simulink model "est_project_cmsd"  (R2022b)
settings: Solver=ode23  StartTime=0.0  StopTime=50  FixedStep=1e-4  MaxStep=0.1  RelTol=1e-6
values from neighbouring files (symbols this model uses):
  A = [0 0 1 0 ... (first row only)    [cmsd_script.m]
  B = [0,0 ... (first row only)    [cmsd_script.m]
  C = [1 0 0 0 ... (first row only)    [cmsd_script.m]
  delta1 = 1/10    (= 0.1)    [cmsd_nonlinear_discrete.m]    (also in cmsd_script.m)
  delta2 = 1/5    (= 0.2)    [cmsd_nonlinear_discrete.m]    (also in cmsd_script.m)
  F = T*A-K1*C    [cmsd_script.m]
  K = place(A,B,[-3,-3,-4,-4])    [cmsd_script.m]
  k1 = 2/5    (= 0.4)    [cmsd_nonlinear_discrete.m]    (also in cmsd_script.m)
  k2 = 1    [cmsd_nonlinear_discrete.m]    (also in cmsd_script.m)
  L = place(A',C',[-10,-10,-20,-20])'    [cmsd_script.m]
  m1 = 1    [cmsd_nonlinear_discrete.m]    (also in cmsd_script.m)
  m2 = 2    [cmsd_nonlinear_discrete.m]    (also in cmsd_script.m)
  miu1 = 1/6    (= 0.166666666667)    [cmsd_nonlinear_discrete.m]    (also in cmsd_script.m)
  miu2 = 1/10    (= 0.1)    [cmsd_nonlinear_discrete.m]    (also in cmsd_script.m)
settings Model: Creator=Alex  LastModifiedBy=Alex

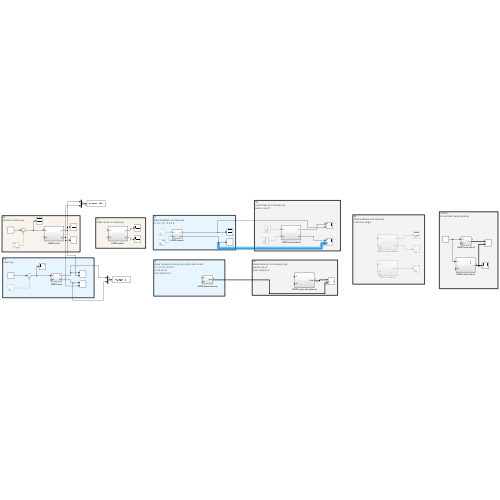
[thumbnail: Simulink's stored preview of the top-level diagram]
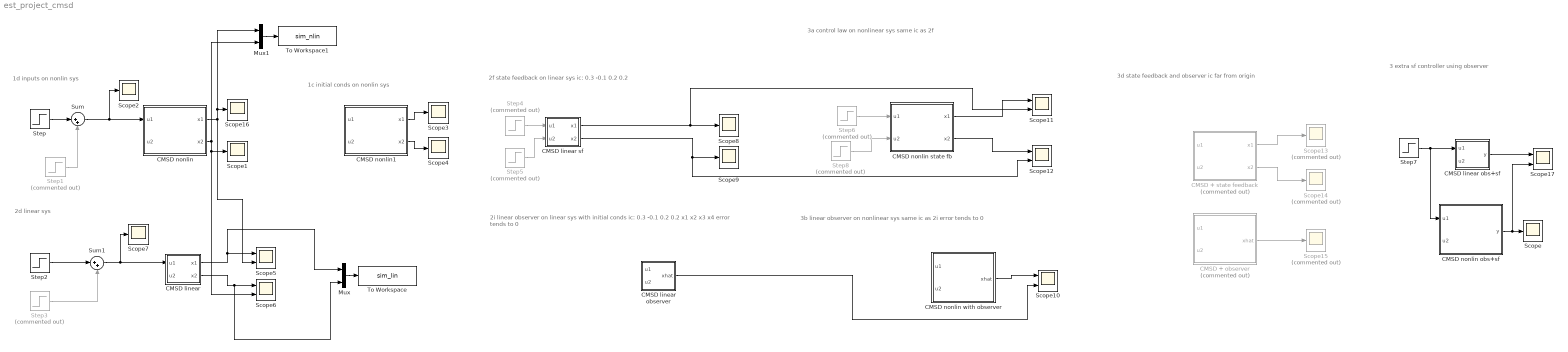
== system est_project_cmsd ==
  note: 3 extra
      | sf controller using observer
  note: 3d
      | state feedback and observer
      | ic far from origin
  note: 3b
      | linear observer on nonlinear sys
      | same ic as 2i
      | error tends to 0
  note: 3a
      | control law on nonlinear sys
      | same ic as 2f
  note: 2i
      | linear observer on linear sys with initial conds
      | ic: 0.3 -0.1 0.2 0.2
      | x1 x2 x3 x4
      | error tends to 0
  note: 2f
      | state feedback on linear sys
      | ic: 0.3 -0.1  0.2 0.2
  note: 2d
      | linear sys
  note: 1d
      | inputs on nonlin sys
  note: 1c
      | initial conds on nonlin sys
  CMSD + observer : Subsystem  Commented=on
  CMSD + state feedback : Subsystem  Commented=on
  CMSD linear : Subsystem
  CMSD linear obs+sf : Subsystem
  CMSD linear observer : Subsystem
  CMSD linear sf : Subsystem
  CMSD nonlin : Subsystem
  CMSD nonlin obs+sf : Subsystem
  CMSD nonlin state fb : Subsystem
  CMSD nonlin with observer : Subsystem
  CMSD nonlin1 : Subsystem
  Mux : Mux  Inputs=2
  Mux1 : Mux  Inputs=2
  Scope{,1..4,7..9,16} (9 alike) : Scope
  Scope{5..6,10..12,17} (6 alike) : Scope  NumInputPorts=2
  Scope13 : Scope  Commented=on
  Scope14 : Scope  Commented=on
  Scope15 : Scope  Commented=on
  Step : Step  Time=0  After=0.1  SampleTime=0
  Step1 : Step  Commented=on  Time=2  After=-0.1  SampleTime=0
  Step2 : Step  Time=0  After=0.1  SampleTime=0
  Step3 : Step  Commented=on  Time=2  After=-0.1  SampleTime=0
  Step4 : Step  Commented=on  SampleTime=0
  Step5 : Step  Commented=on  After=0.2  SampleTime=0
  Step6 : Step  Commented=on  SampleTime=0
  Step7 : Step  After=5  SampleTime=0
  Step8 : Step  Commented=on  After=0.2  SampleTime=0
  Sum : Sum  Inputs=|++
  Sum1 : Sum  Inputs=|++
  To Workspace : ToWorkspace  VariableName=sim_lin  SampleTime=-1
  To Workspace1 : ToWorkspace  VariableName=sim_nlin  SampleTime=-1
  wires:
  Step/1 -> Sum/1
  Step1/1 -> Sum/2
  Sum/1 -> Scope2/1, CMSD nonlin/1(u1)
  CMSD nonlin1/2(x2) -> Scope4/1
  CMSD nonlin1/1(x1) -> Scope3/1
  Sum1/1 -> Scope7/1, CMSD linear/1(u1)
  Step3/1 -> Sum1/2
  Step2/1 -> Sum1/1
  CMSD linear sf/2(x2) -> Scope12/2, Scope9/1
  CMSD linear sf/1(x1) -> Scope11/2, Scope8/1
  CMSD nonlin state fb/1(x1) -> Scope11/1
  CMSD nonlin state fb/2(x2) -> Scope12/1
  CMSD nonlin with observer/1(xhat) -> Scope10/1
  CMSD linear observer/1(xhat) -> Scope10/2
  CMSD + state feedback/1(x1) -> Scope13/1
  CMSD + state feedback/2(x2) -> Scope14/1
  CMSD + observer/1(xhat) -> Scope15/1
  Step4/1 -> CMSD linear sf/1(u1)
  Step5/1 -> CMSD linear sf/2(u2)
  Step6/1 -> CMSD nonlin state fb/1(u1)
  CMSD linear/1(x1) -> Mux/1, Scope5/1
  CMSD nonlin/1(x1) -> Mux1/1, Scope16/1, Scope5/2
  CMSD linear/2(x2) -> Mux/2, Scope6/1
  CMSD nonlin/2(x2) -> Mux1/2, Scope1/1, Scope6/2
  CMSD nonlin obs+sf/1(y) -> Scope17/2, Scope/1
  CMSD linear obs+sf/1(y) -> Scope17/1
  Step7/1 -> CMSD nonlin obs+sf/1(u1), CMSD linear obs+sf/1(u1)
  Step8/1 -> CMSD nonlin state fb/2(u2)
  Mux/1 -> To Workspace/1
  Mux1/1 -> To Workspace1/1

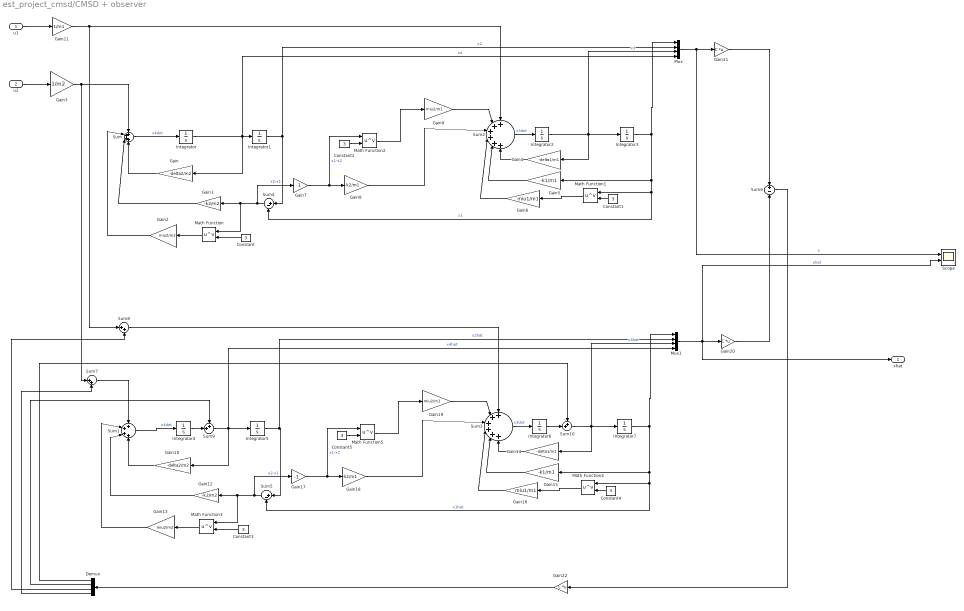
== system est_project_cmsd/CMSD + observer ==
  u1 : Inport
  u2 : Inport  Port=2
  Constant{,1..5} (6 alike) : Constant  Value=3
  Demux : Demux
  Gain : Gain  Gain=-delta2/m2
  Gain1 : Gain  Gain=-k2/m2
  Gain10 : Gain  Gain=-delta2/m2
  Gain11 : Gain  Gain=1/m1
  Gain12 : Gain  Gain=-k2/m2
  Gain13 : Gain  Gain=miu2/m2
  Gain14 : Gain  Gain=-delta1/m1
  Gain15 : Gain  Gain=-k1/m1
  Gain16 : Gain  Gain=miu1/m1
  Gain17 : Gain  Gain=-1
  Gain18 : Gain  Gain=-k2/m1
  Gain19 : Gain  Gain=miu2/m1
  Gain2 : Gain  Gain=miu2/m2
  Gain20 : Gain  Gain=C  Multiplication=Matrix(K*u)
  Gain21 : Gain  Gain=C  Multiplication=Matrix(K*u)
  Gain22 : Gain  Gain=L  Multiplication=Matrix(K*u)
  Gain3 : Gain  Gain=1/m2
  Gain4 : Gain  Gain=-delta1/m1
  Gain5 : Gain  Gain=-k1/m1
  Gain6 : Gain  Gain=miu1/m1
  Gain7 : Gain  Gain=-1
  Gain8 : Gain  Gain=-k2/m1
  Gain9 : Gain  Gain=miu2/m1
  Integrator : Integrator  InitialCondition=0.7
  Integrator1 : Integrator  InitialCondition=-0.6
  Integrator2 : Integrator  InitialCondition=-0.7
  Integrator3 : Integrator  InitialCondition=0.5
  Integrator{4..7} (4 alike) : Integrator
  Math Function{,1..5} (6 alike) : Math  Operator=pow
  Mux : Mux
  Mux1 : Mux
  Scope : Scope  NumInputPorts=2
  Sum : Sum  Inputs=++++
  Sum1 : Sum  Inputs=++++
  Sum10 : Sum  Inputs=++|
  Sum2 : Sum  Inputs=++++++
  Sum3 : Sum  Inputs=++++++
  Sum4 : Sum  Inputs=|+-
  Sum5 : Sum  Inputs=|+-
  Sum6 : Sum  Inputs=+-
  Sum7 : Sum  Inputs=|++
  Sum8 : Sum  Inputs=|++
  Sum9 : Sum  Inputs=++|
  xhat : Outport
  wires:
  Demux/1 -> Sum10/1
  Sum10/1 -> Integrator7/1, Gain14/1, Mux1/3  "x3hat"
  Integrator6/1 -> Sum10/2
  Demux/2 -> Sum9/1
  Sum9/1 -> Integrator5/1, Gain10/1, Mux1/4  "x4hat"
  Integrator4/1 -> Sum9/2
  Demux/3 -> Sum8/2
  Demux/4 -> Sum7/2
  Sum8/1 -> Sum3/1
  Sum7/1 -> Sum1/1
  Gain22/1 -> Demux/1
  Sum6/1 -> Gain22/1
  Gain21/1 -> Sum6/1
  Gain20/1 -> Sum6/2
  Mux1/1 -> Gain20/1, Scope/2, xhat/1  "xhat"
  Gain14/1 -> Sum3/6
  Sum5/1 -> Gain17/1, Math Function3/1, Gain12/1  "x2-x1"
  Integrator7/1 -> Sum5/2, Math Function4/1, Gain15/1, Mux1/1  "x1hat"
  Gain18/1 -> Sum3/3
  Gain17/1 -> Math Function5/1, Gain18/1  "x1-x2"
  Math Function5/1 -> Gain19/1
  Gain15/1 -> Sum3/5
  Gain12/1 -> Sum1/3
  Constant5/1 -> Math Function5/2
  Gain19/1 -> Sum3/2
  Sum1/1 -> Integrator4/1  "x4dot"
  Math Function4/1 -> Gain16/1
  Gain10/1 -> Sum1/4
  Gain13/1 -> Sum1/2
  Integrator5/1 -> Mux1/2, Sum5/1  "x2hat"
  Constant3/1 -> Math Function3/2
  Math Function3/1 -> Gain13/1
  Gain16/1 -> Sum3/4
  Sum3/1 -> Integrator6/1  "x3dot"
  Constant4/1 -> Math Function4/2
  Gain11/1 -> Sum2/1, Sum8/1
  Constant1/1 -> Math Function1/2
  Sum2/1 -> Integrator2/1  "x3dot"
  u2/1 -> Gain3/1
  Gain6/1 -> Sum2/4
  Integrator2/1 -> Mux/3, Integrator3/1, Gain4/1  "x3"
  Math Function/1 -> Gain2/1
  Constant/1 -> Math Function/2
  Integrator1/1 -> Sum4/1, Mux/2  "x2"
  Gain2/1 -> Sum/2
  Gain/1 -> Sum/4
  Math Function1/1 -> Gain6/1
  Sum/1 -> Integrator/1  "x4dot"
  Gain9/1 -> Sum2/2
  Constant2/1 -> Math Function2/2
  Gain1/1 -> Sum/3
  Gain5/1 -> Sum2/5
  Math Function2/1 -> Gain9/1
  Gain7/1 -> Gain8/1, Math Function2/1  "x1-x2"
  Gain8/1 -> Sum2/3
  Integrator3/1 -> Mux/1, Gain5/1, Math Function1/1, Sum4/2  "x1"
  Sum4/1 -> Gain1/1, Math Function/1, Gain7/1  "x2-x1"
  Integrator/1 -> Mux/4, Integrator1/1, Gain/1  "x4"
  Gain4/1 -> Sum2/6
  Mux/1 -> Gain21/1, Scope/1  "x"
  Gain3/1 -> Sum/1, Sum7/1
  u1/1 -> Gain11/1

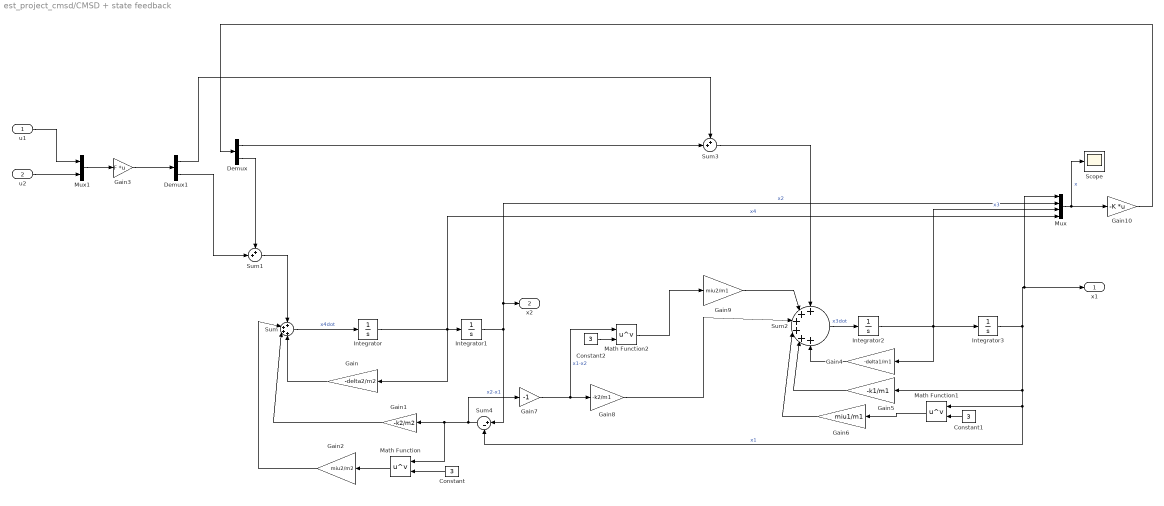
== system est_project_cmsd/CMSD + state feedback ==
  u1 : Inport
  u2 : Inport  Port=2
  Constant : Constant  Value=3
  Constant1 : Constant  Value=3
  Constant2 : Constant  Value=3
  Demux : Demux  Outputs=2
  Demux1 : Demux  Outputs=2
  Gain : Gain  Gain=-delta2/m2
  Gain1 : Gain  Gain=-k2/m2
  Gain10 : Gain  Gain=-K  Multiplication=Matrix(K*u)
  Gain2 : Gain  Gain=miu2/m2
  Gain3 : Gain  Gain=F  Multiplication=Matrix(K*u)
  Gain4 : Gain  Gain=-delta1/m1
  Gain5 : Gain  Gain=-k1/m1
  Gain6 : Gain  Gain=miu1/m1
  Gain7 : Gain  Gain=-1
  Gain8 : Gain  Gain=-k2/m1
  Gain9 : Gain  Gain=miu2/m1
  Integrator{,1..3} (4 alike) : Integrator  InitialCondition=1
  Math Function : Math  Operator=pow
  Math Function1 : Math  Operator=pow
  Math Function2 : Math  Operator=pow
  Mux : Mux
  Mux1 : Mux  Inputs=2
  Scope : Scope
  Sum : Sum  Inputs=++++
  Sum1 : Sum  Inputs=++|
  Sum2 : Sum  Inputs=++++++
  Sum3 : Sum  Inputs=++|
  Sum4 : Sum  Inputs=|+-
  x1 : Outport
  x2 : Outport  Port=2
  wires:
  Sum3/1 -> Sum2/1
  Demux/1 -> Sum3/2
  Sum1/1 -> Sum/1
  Demux/2 -> Sum1/1
  Gain10/1 -> Demux/1
  Mux/1 -> Gain10/1, Scope/1  "x"
  Gain4/1 -> Sum2/6
  Integrator/1 -> Gain/1, Integrator1/1, Mux/4  "x4"
  Sum4/1 -> Gain7/1, Math Function/1, Gain1/1  "x2-x1"
  Integrator3/1 -> Sum4/2, Math Function1/1, Gain5/1, x1/1, Mux/1  "x1"
  Gain8/1 -> Sum2/3
  Gain7/1 -> Math Function2/1, Gain8/1  "x1-x2"
  Math Function2/1 -> Gain9/1
  Gain5/1 -> Sum2/5
  Gain1/1 -> Sum/3
  Constant2/1 -> Math Function2/2
  Gain9/1 -> Sum2/2
  Sum/1 -> Integrator/1  "x4dot"
  Math Function1/1 -> Gain6/1
  Gain/1 -> Sum/4
  Gain2/1 -> Sum/2
  Integrator1/1 -> x2/1, Mux/2, Sum4/1  "x2"
  Constant/1 -> Math Function/2
  Math Function/1 -> Gain2/1
  Integrator2/1 -> Gain4/1, Integrator3/1, Mux/3  "x3"
  Gain6/1 -> Sum2/4
  Sum2/1 -> Integrator2/1  "x3dot"
  Constant1/1 -> Math Function1/2
  u1/1 -> Mux1/1
  u2/1 -> Mux1/2
  Mux1/1 -> Gain3/1
  Gain3/1 -> Demux1/1
  Demux1/1 -> Sum3/1
  Demux1/2 -> Sum1/2

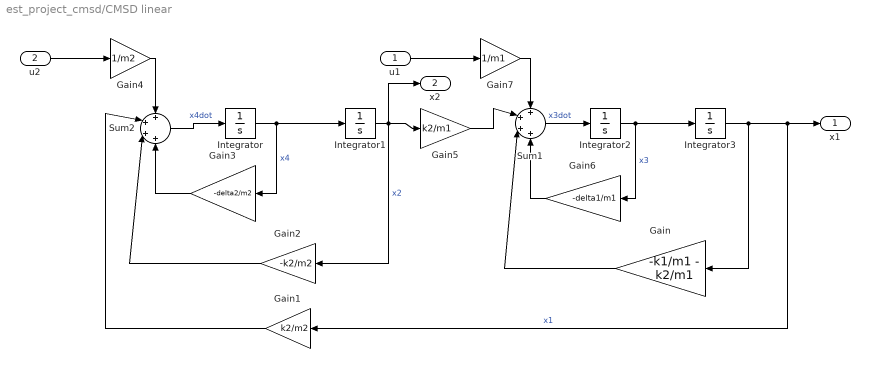
== system est_project_cmsd/CMSD linear ==
  u1 : Inport
  u2 : Inport  Port=2
  Gain : Gain  Gain=-k1/m1 - k2/m1
  Gain1 : Gain  Gain=k2/m2
  Gain2 : Gain  Gain=-k2/m2
  Gain3 : Gain  Gain=-delta2/m2
  Gain4 : Gain  Gain=1/m2
  Gain5 : Gain  Gain=k2/m1
  Gain6 : Gain  Gain=-delta1/m1
  Gain7 : Gain  Gain=1/m1
  Integrator{,1..3} (4 alike) : Integrator
  Sum1 : Sum  Inputs=++++
  Sum2 : Sum  Inputs=++++
  x1 : Outport
  x2 : Outport  Port=2
  wires:
  Integrator1/1 -> Gain2/1, Gain5/1, x2/1  "x2"
  Gain6/1 -> Sum1/4
  Gain/1 -> Sum1/3
  u2/1 -> Gain4/1
  Integrator3/1 -> Gain/1, x1/1, Gain1/1  "x1"
  Integrator/1 -> Gain3/1, Integrator1/1  "x4"
  Gain5/1 -> Sum1/2
  Gain7/1 -> Sum1/1
  Gain4/1 -> Sum2/1
  Sum2/1 -> Integrator/1  "x4dot"
  Sum1/1 -> Integrator2/1  "x3dot"
  Integrator2/1 -> Gain6/1, Integrator3/1  "x3"
  u1/1 -> Gain7/1
  Gain2/1 -> Sum2/3
  Gain1/1 -> Sum2/2
  Gain3/1 -> Sum2/4

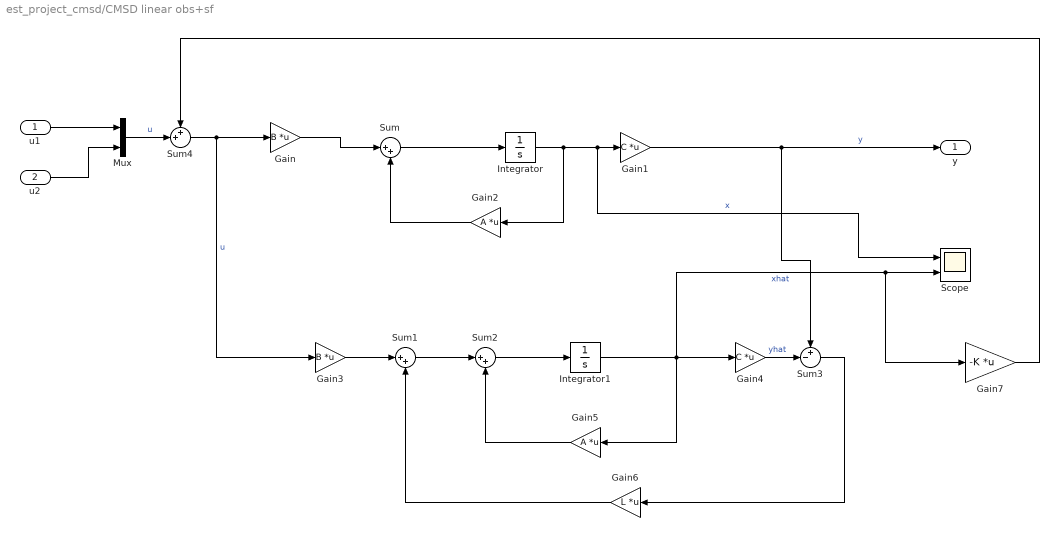
== system est_project_cmsd/CMSD linear obs+sf ==
  u1 : Inport
  u2 : Inport  Port=2
  Gain : Gain  Gain=B  Multiplication=Matrix(K*u)
  Gain1 : Gain  Gain=C  Multiplication=Matrix(K*u)
  Gain2 : Gain  Gain=A  Multiplication=Matrix(K*u)
  Gain3 : Gain  Gain=B  Multiplication=Matrix(K*u)
  Gain4 : Gain  Gain=C  Multiplication=Matrix(K*u)
  Gain5 : Gain  Gain=A  Multiplication=Matrix(K*u)
  Gain6 : Gain  Gain=L  Multiplication=Matrix(K*u)
  Gain7 : Gain  Gain=-K  Multiplication=Matrix(K*u)
  Integrator : Integrator  InitialCondition=[0.3 -0.1 0.2 0.2]
  Integrator1 : Integrator
  Mux : Mux  Inputs=2
  Scope : Scope  NumInputPorts=2
  Sum : Sum  Inputs=|++
  Sum1 : Sum  Inputs=|++
  Sum2 : Sum  Inputs=|++
  Sum3 : Sum  Inputs=+-|
  Sum4 : Sum  Inputs=++|
  y : Outport
  wires:
  Gain6/1 -> Sum1/2
  Sum3/1 -> Gain6/1
  Gain4/1 -> Sum3/2  "yhat"
  Gain5/1 -> Sum2/2
  Integrator1/1 -> Gain4/1, Gain5/1, Gain7/1, Scope/2  "xhat"
  Sum2/1 -> Integrator1/1
  Sum1/1 -> Sum2/1
  Gain3/1 -> Sum1/1
  Gain1/1 -> Sum3/1, y/1  "y"
  Gain2/1 -> Sum/2
  Integrator/1 -> Gain1/1, Scope/1, Gain2/1  "x"
  Sum/1 -> Integrator/1
  Gain/1 -> Sum/1
  u2/1 -> Mux/2
  u1/1 -> Mux/1
  Gain7/1 -> Sum4/1
  Mux/1 -> Sum4/2  "u"
  Sum4/1 -> Gain3/1, Gain/1  "u"

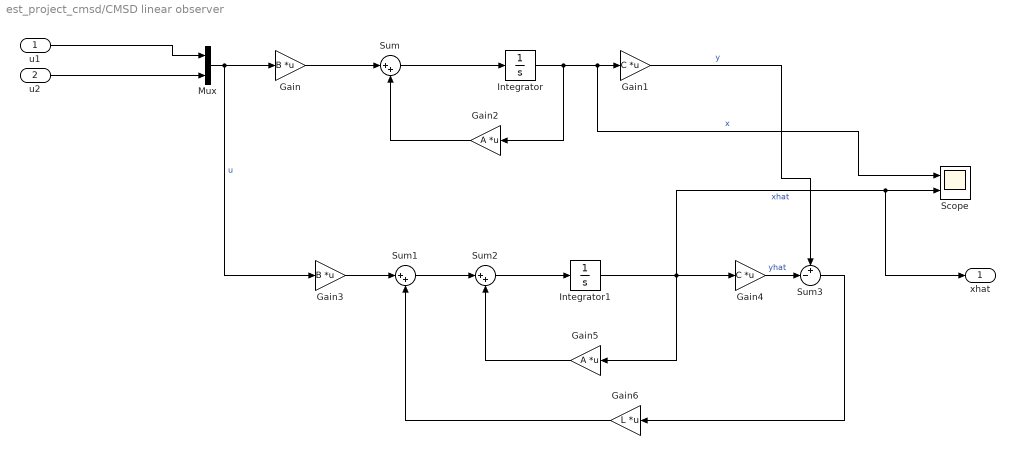
== system est_project_cmsd/CMSD linear observer ==
  u1 : Inport
  u2 : Inport  Port=2
  Gain : Gain  Gain=B  Multiplication=Matrix(K*u)
  Gain1 : Gain  Gain=C  Multiplication=Matrix(K*u)
  Gain2 : Gain  Gain=A  Multiplication=Matrix(K*u)
  Gain3 : Gain  Gain=B  Multiplication=Matrix(K*u)
  Gain4 : Gain  Gain=C  Multiplication=Matrix(K*u)
  Gain5 : Gain  Gain=A  Multiplication=Matrix(K*u)
  Gain6 : Gain  Gain=L  Multiplication=Matrix(K*u)
  Integrator : Integrator  InitialCondition=[0.3 -0.1 0.2 0.2]
  Integrator1 : Integrator
  Mux : Mux  Inputs=2
  Scope : Scope  NumInputPorts=2
  Sum : Sum  Inputs=|++
  Sum1 : Sum  Inputs=|++
  Sum2 : Sum  Inputs=|++
  Sum3 : Sum  Inputs=+-|
  xhat : Outport
  wires:
  u1/1 -> Mux/1
  u2/1 -> Mux/2
  Mux/1 -> Gain3/1, Gain/1  "u"
  Gain/1 -> Sum/1
  Sum/1 -> Integrator/1
  Integrator/1 -> Gain2/1, Scope/1, Gain1/1  "x"
  Gain2/1 -> Sum/2
  Gain1/1 -> Sum3/1  "y"
  Gain3/1 -> Sum1/1
  Sum1/1 -> Sum2/1
  Sum2/1 -> Integrator1/1
  Integrator1/1 -> xhat/1, Scope/2, Gain5/1, Gain4/1  "xhat"
  Gain5/1 -> Sum2/2
  Gain4/1 -> Sum3/2  "yhat"
  Sum3/1 -> Gain6/1
  Gain6/1 -> Sum1/2

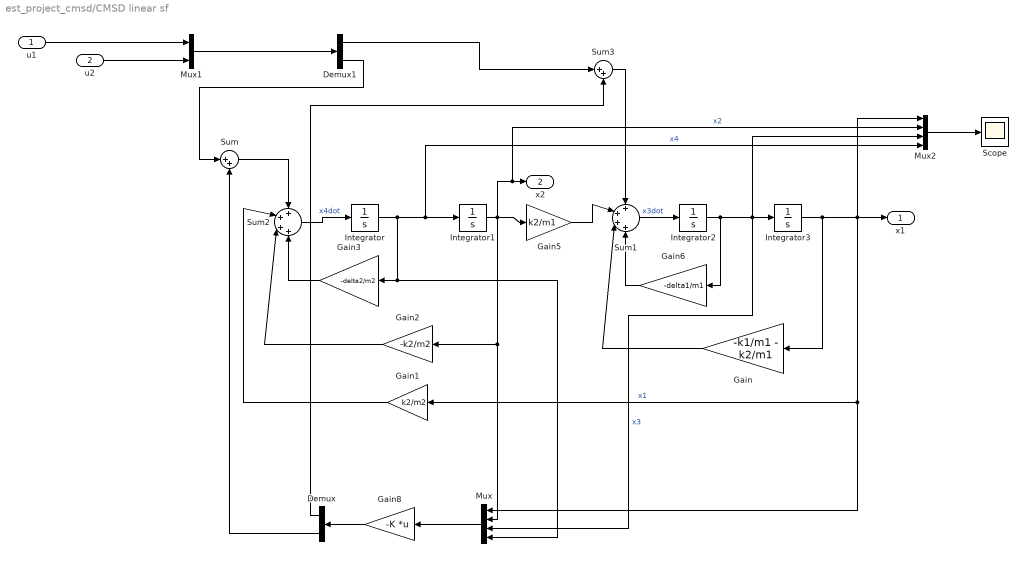
== system est_project_cmsd/CMSD linear sf ==
  u1 : Inport
  u2 : Inport  Port=2
  Demux : Demux  Outputs=2
  Demux1 : Demux  Outputs=2
  Gain : Gain  Gain=-k1/m1 - k2/m1
  Gain1 : Gain  Gain=k2/m2
  Gain2 : Gain  Gain=-k2/m2
  Gain3 : Gain  Gain=-delta2/m2
  Gain5 : Gain  Gain=k2/m1
  Gain6 : Gain  Gain=-delta1/m1
  Gain8 : Gain  Gain=-K  Multiplication=Matrix(K*u)
  Integrator : Integrator  InitialCondition=0.2
  Integrator1 : Integrator  InitialCondition=-0.1
  Integrator2 : Integrator  InitialCondition=0.2
  Integrator3 : Integrator  InitialCondition=0.3
  Mux : Mux
  Mux1 : Mux  Inputs=2
  Mux2 : Mux
  Scope : Scope
  Sum : Sum  Inputs=|++
  Sum1 : Sum  Inputs=++++
  Sum2 : Sum  Inputs=++++
  Sum3 : Sum  Inputs=|++
  x1 : Outport
  x2 : Outport  Port=2
  wires:
  Gain3/1 -> Sum2/4
  Gain1/1 -> Sum2/2
  Gain2/1 -> Sum2/3
  Integrator2/1 -> Mux2/3, Mux/3, Integrator3/1, Gain6/1  "x3"
  Sum1/1 -> Integrator2/1  "x3dot"
  Sum2/1 -> Integrator/1  "x4dot"
  Gain5/1 -> Sum1/2
  Integrator/1 -> Mux2/4, Integrator1/1, Mux/4, Gain3/1  "x4"
  Integrator3/1 -> Mux2/1, Mux/1, Gain1/1, x1/1, Gain/1  "x1"
  Gain/1 -> Sum1/3
  Gain6/1 -> Sum1/4
  Integrator1/1 -> Mux2/2, x2/1, Gain5/1, Gain2/1, Mux/2  "x2"
  Mux/1 -> Gain8/1
  Gain8/1 -> Demux/1
  Demux/1 -> Sum3/2
  Demux/2 -> Sum/2
  Sum/1 -> Sum2/1
  Sum3/1 -> Sum1/1
  u1/1 -> Mux1/1
  u2/1 -> Mux1/2
  Mux1/1 -> Demux1/1
  Demux1/2 -> Sum/1
  Demux1/1 -> Sum3/1
  Mux2/1 -> Scope/1

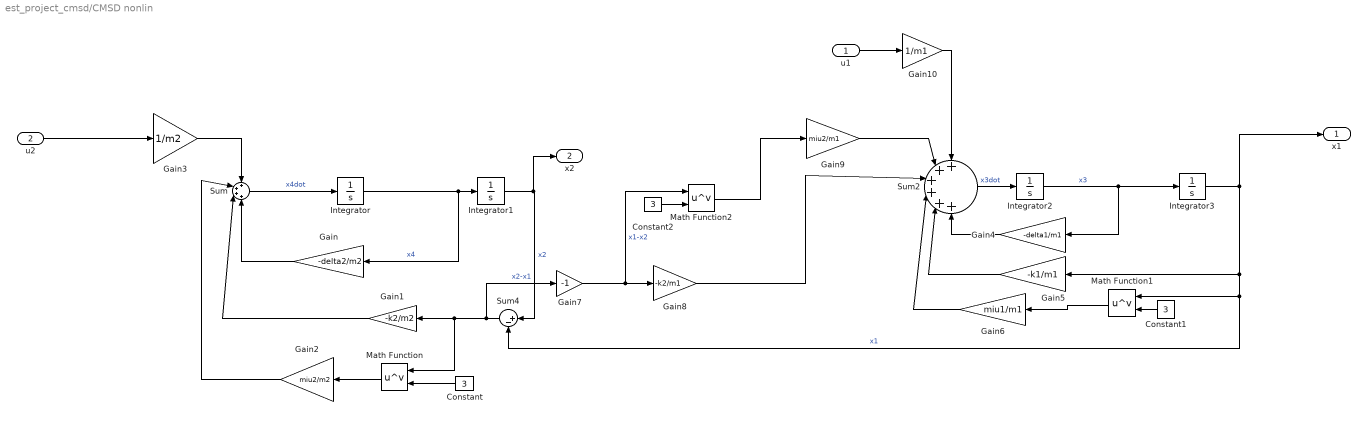
== system est_project_cmsd/CMSD nonlin ==
  u1 : Inport
  u2 : Inport  Port=2
  Constant : Constant  Value=3
  Constant1 : Constant  Value=3
  Constant2 : Constant  Value=3
  Gain : Gain  Gain=-delta2/m2
  Gain1 : Gain  Gain=-k2/m2
  Gain10 : Gain  Gain=1/m1
  Gain2 : Gain  Gain=miu2/m2
  Gain3 : Gain  Gain=1/m2
  Gain4 : Gain  Gain=-delta1/m1
  Gain5 : Gain  Gain=-k1/m1
  Gain6 : Gain  Gain=miu1/m1
  Gain7 : Gain  Gain=-1
  Gain8 : Gain  Gain=-k2/m1
  Gain9 : Gain  Gain=miu2/m1
  Integrator{,1..3} (4 alike) : Integrator
  Math Function : Math  Operator=pow
  Math Function1 : Math  Operator=pow
  Math Function2 : Math  Operator=pow
  Sum : Sum  Inputs=++++
  Sum2 : Sum  Inputs=++++++
  Sum4 : Sum  Inputs=|+-
  x1 : Outport
  x2 : Outport  Port=2
  wires:
  Gain4/1 -> Sum2/6
  Integrator/1 -> Gain/1, Integrator1/1  "x4"
  Sum4/1 -> Gain7/1, Math Function/1, Gain1/1  "x2-x1"
  Integrator3/1 -> Sum4/2, Math Function1/1, Gain5/1, x1/1  "x1"
  Gain8/1 -> Sum2/3
  Gain7/1 -> Math Function2/1, Gain8/1  "x1-x2"
  Math Function2/1 -> Gain9/1
  Gain3/1 -> Sum/1
  Gain5/1 -> Sum2/5
  Gain1/1 -> Sum/3
  Constant2/1 -> Math Function2/2
  Gain9/1 -> Sum2/2
  Sum/1 -> Integrator/1  "x4dot"
  Math Function1/1 -> Gain6/1
  Gain/1 -> Sum/4
  Gain2/1 -> Sum/2
  Integrator1/1 -> x2/1, Sum4/1  "x2"
  Constant/1 -> Math Function/2
  Math Function/1 -> Gain2/1
  Integrator2/1 -> Gain4/1, Integrator3/1  "x3"
  Gain6/1 -> Sum2/4
  u2/1 -> Gain3/1
  Sum2/1 -> Integrator2/1  "x3dot"
  Constant1/1 -> Math Function1/2
  u1/1 -> Gain10/1
  Gain10/1 -> Sum2/1

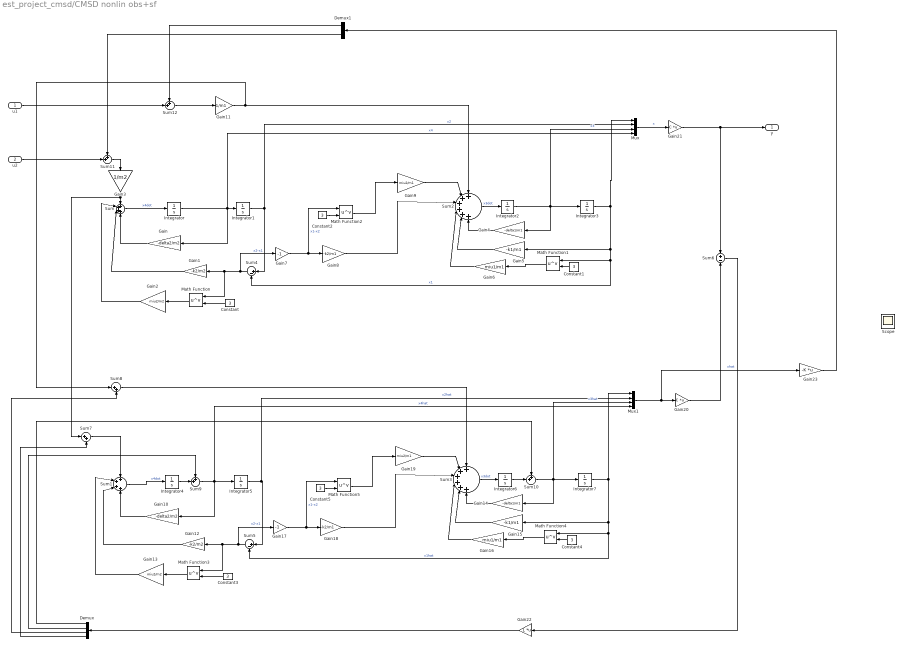
== system est_project_cmsd/CMSD nonlin obs+sf ==
  u1 : Inport
  u2 : Inport  Port=2
  Constant{,1..5} (6 alike) : Constant  Value=3
  Demux : Demux
  Demux1 : Demux  Outputs=2
  Gain : Gain  Gain=-delta2/m2
  Gain1 : Gain  Gain=-k2/m2
  Gain10 : Gain  Gain=-delta2/m2
  Gain11 : Gain  Gain=1/m1
  Gain12 : Gain  Gain=-k2/m2
  Gain13 : Gain  Gain=miu2/m2
  Gain14 : Gain  Gain=-delta1/m1
  Gain15 : Gain  Gain=-k1/m1
  Gain16 : Gain  Gain=miu1/m1
  Gain17 : Gain  Gain=-1
  Gain18 : Gain  Gain=-k2/m1
  Gain19 : Gain  Gain=miu2/m1
  Gain2 : Gain  Gain=miu2/m2
  Gain20 : Gain  Gain=C  Multiplication=Matrix(K*u)
  Gain21 : Gain  Gain=C  Multiplication=Matrix(K*u)
  Gain22 : Gain  Gain=L  Multiplication=Matrix(K*u)
  Gain23 : Gain  Gain=-K  Multiplication=Matrix(K*u)
  Gain3 : Gain  Gain=1/m2
  Gain4 : Gain  Gain=-delta1/m1
  Gain5 : Gain  Gain=-k1/m1
  Gain6 : Gain  Gain=miu1/m1
  Gain7 : Gain  Gain=-1
  Gain8 : Gain  Gain=-k2/m1
  Gain9 : Gain  Gain=miu2/m1
  Integrator : Integrator  InitialCondition=0.2
  Integrator1 : Integrator  InitialCondition=-0.1
  Integrator2 : Integrator  InitialCondition=0.2
  Integrator3 : Integrator  InitialCondition=0.3
  Integrator{4..7} (4 alike) : Integrator
  Math Function{,1..5} (6 alike) : Math  Operator=pow
  Mux : Mux
  Mux1 : Mux
  Scope : Scope  NumInputPorts=2
  Sum : Sum  Inputs=++++
  Sum1 : Sum  Inputs=++++
  Sum{9..12} (4 alike) : Sum  Inputs=++|
  Sum2 : Sum  Inputs=++++++
  Sum3 : Sum  Inputs=++++++
  Sum4 : Sum  Inputs=|+-
  Sum5 : Sum  Inputs=|+-
  Sum6 : Sum  Inputs=+-
  Sum7 : Sum  Inputs=|++
  Sum8 : Sum  Inputs=|++
  y : Outport
  wires:
  Demux/1 -> Sum10/1
  Sum10/1 -> Integrator7/1, Gain14/1, Mux1/3  "x3hat"
  Integrator6/1 -> Sum10/2
  Demux/2 -> Sum9/1
  Sum9/1 -> Integrator5/1, Gain10/1, Mux1/4  "x4hat"
  Integrator4/1 -> Sum9/2
  Demux/3 -> Sum8/2
  Demux/4 -> Sum7/2
  Sum8/1 -> Sum3/1
  Sum7/1 -> Sum1/1
  Gain22/1 -> Demux/1
  Sum6/1 -> Gain22/1
  Gain21/1 -> y/1, Sum6/1
  Gain20/1 -> Sum6/2
  Mux1/1 -> Gain23/1, Gain20/1  "xhat"
  Gain14/1 -> Sum3/6
  Sum5/1 -> Gain17/1, Math Function3/1, Gain12/1  "x2-x1"
  Integrator7/1 -> Sum5/2, Math Function4/1, Gain15/1, Mux1/1  "x1hat"
  Gain18/1 -> Sum3/3
  Gain17/1 -> Math Function5/1, Gain18/1  "x1-x2"
  Math Function5/1 -> Gain19/1
  Gain15/1 -> Sum3/5
  Gain12/1 -> Sum1/3
  Constant5/1 -> Math Function5/2
  Gain19/1 -> Sum3/2
  Sum1/1 -> Integrator4/1  "x4dot"
  Math Function4/1 -> Gain16/1
  Gain10/1 -> Sum1/4
  Gain13/1 -> Sum1/2
  Integrator5/1 -> Mux1/2, Sum5/1  "x2hat"
  Constant3/1 -> Math Function3/2
  Math Function3/1 -> Gain13/1
  Gain16/1 -> Sum3/4
  Sum3/1 -> Integrator6/1  "x3dot"
  Constant4/1 -> Math Function4/2
  u1/1 -> Sum12/2
  Constant1/1 -> Math Function1/2
  Sum2/1 -> Integrator2/1  "x3dot"
  Gain6/1 -> Sum2/4
  Integrator2/1 -> Mux/3, Integrator3/1, Gain4/1  "x3"
  Math Function/1 -> Gain2/1
  Constant/1 -> Math Function/2
  Integrator1/1 -> Sum4/1, Mux/2  "x2"
  Gain2/1 -> Sum/2
  Gain/1 -> Sum/4
  Math Function1/1 -> Gain6/1
  Sum/1 -> Integrator/1  "x4dot"
  Gain9/1 -> Sum2/2
  Constant2/1 -> Math Function2/2
  Gain1/1 -> Sum/3
  Gain5/1 -> Sum2/5
  Math Function2/1 -> Gain9/1
  Gain7/1 -> Gain8/1, Math Function2/1  "x1-x2"
  Gain8/1 -> Sum2/3
  Integrator3/1 -> Mux/1, Gain5/1, Math Function1/1, Sum4/2  "x1"
  Sum4/1 -> Gain1/1, Math Function/1, Gain7/1  "x2-x1"
  Integrator/1 -> Mux/4, Integrator1/1, Gain/1  "x4"
  Gain4/1 -> Sum2/6
  Mux/1 -> Gain21/1  "x"
  u2/1 -> Sum11/2
  Gain23/1 -> Demux1/1
  Sum11/1 -> Gain3/1
  Demux1/2 -> Sum11/1
  Sum12/1 -> Gain11/1
  Demux1/1 -> Sum12/1
  Gain3/1 -> Sum7/1, Sum/1
  Gain11/1 -> Sum8/1, Sum2/1

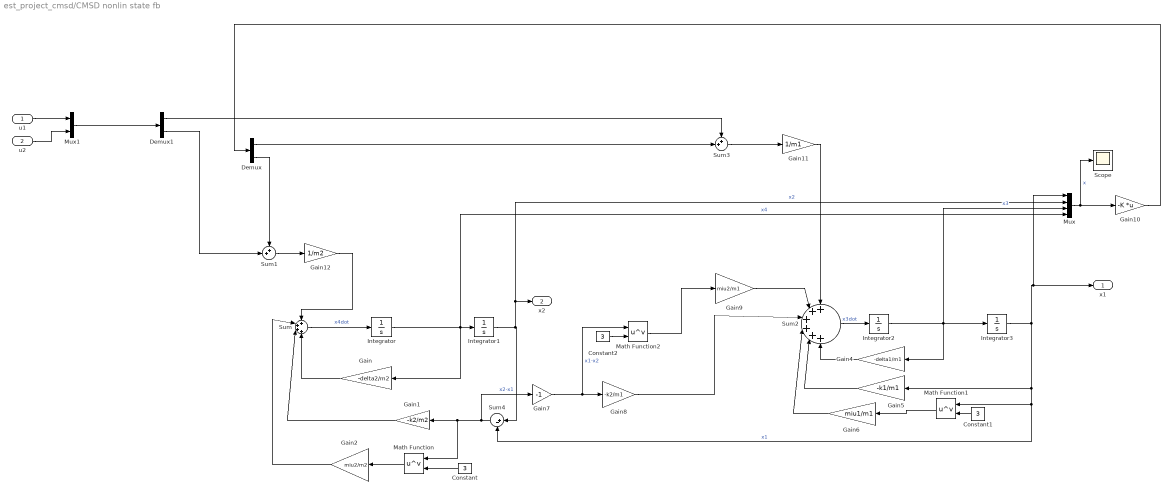
== system est_project_cmsd/CMSD nonlin state fb ==
  u1 : Inport
  u2 : Inport  Port=2
  Constant : Constant  Value=3
  Constant1 : Constant  Value=3
  Constant2 : Constant  Value=3
  Demux : Demux  Outputs=2
  Demux1 : Demux  Outputs=2
  Gain : Gain  Gain=-delta2/m2
  Gain1 : Gain  Gain=-k2/m2
  Gain10 : Gain  Gain=-K  Multiplication=Matrix(K*u)
  Gain11 : Gain  Gain=1/m1
  Gain12 : Gain  Gain=1/m2
  Gain2 : Gain  Gain=miu2/m2
  Gain4 : Gain  Gain=-delta1/m1
  Gain5 : Gain  Gain=-k1/m1
  Gain6 : Gain  Gain=miu1/m1
  Gain7 : Gain  Gain=-1
  Gain8 : Gain  Gain=-k2/m1
  Gain9 : Gain  Gain=miu2/m1
  Integrator : Integrator  InitialCondition=0.2
  Integrator1 : Integrator  InitialCondition=-0.1
  Integrator2 : Integrator  InitialCondition=0.2
  Integrator3 : Integrator  InitialCondition=0.3
  Math Function : Math  Operator=pow
  Math Function1 : Math  Operator=pow
  Math Function2 : Math  Operator=pow
  Mux : Mux
  Mux1 : Mux  Inputs=2
  Scope : Scope
  Sum : Sum  Inputs=++++
  Sum1 : Sum  Inputs=++|
  Sum2 : Sum  Inputs=++++++
  Sum3 : Sum  Inputs=++|
  Sum4 : Sum  Inputs=|+-
  x1 : Outport
  x2 : Outport  Port=2
  wires:
  Constant1/1 -> Math Function1/2
  Sum2/1 -> Integrator2/1  "x3dot"
  Gain6/1 -> Sum2/4
  Integrator2/1 -> Mux/3, Integrator3/1, Gain4/1  "x3"
  Math Function/1 -> Gain2/1
  Constant/1 -> Math Function/2
  Integrator1/1 -> Sum4/1, Mux/2, x2/1  "x2"
  Gain2/1 -> Sum/2
  Gain/1 -> Sum/4
  Math Function1/1 -> Gain6/1
  Sum/1 -> Integrator/1  "x4dot"
  Gain9/1 -> Sum2/2
  Constant2/1 -> Math Function2/2
  Gain1/1 -> Sum/3
  Gain5/1 -> Sum2/5
  Math Function2/1 -> Gain9/1
  Gain7/1 -> Gain8/1, Math Function2/1  "x1-x2"
  Gain8/1 -> Sum2/3
  Integrator3/1 -> Mux/1, x1/1, Gain5/1, Math Function1/1, Sum4/2  "x1"
  Sum4/1 -> Gain1/1, Math Function/1, Gain7/1  "x2-x1"
  Integrator/1 -> Mux/4, Integrator1/1, Gain/1  "x4"
  Gain4/1 -> Sum2/6
  Mux/1 -> Scope/1, Gain10/1  "x"
  Gain10/1 -> Demux/1
  Demux/2 -> Sum1/1
  Sum1/1 -> Gain12/1
  Demux/1 -> Sum3/2
  Sum3/1 -> Gain11/1
  u1/1 -> Mux1/1
  u2/1 -> Mux1/2
  Mux1/1 -> Demux1/1
  Demux1/1 -> Sum3/1
  Demux1/2 -> Sum1/2
  Gain11/1 -> Sum2/1
  Gain12/1 -> Sum/1

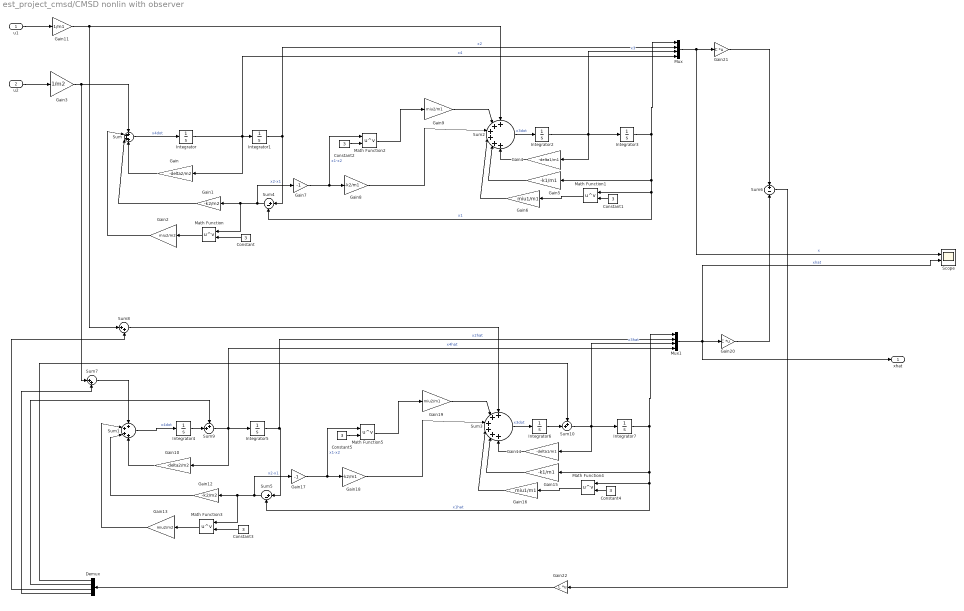
== system est_project_cmsd/CMSD nonlin with observer ==
  u1 : Inport
  u2 : Inport  Port=2
  Constant{,1..5} (6 alike) : Constant  Value=3
  Demux : Demux
  Gain : Gain  Gain=-delta2/m2
  Gain1 : Gain  Gain=-k2/m2
  Gain10 : Gain  Gain=-delta2/m2
  Gain11 : Gain  Gain=1/m1
  Gain12 : Gain  Gain=-k2/m2
  Gain13 : Gain  Gain=miu2/m2
  Gain14 : Gain  Gain=-delta1/m1
  Gain15 : Gain  Gain=-k1/m1
  Gain16 : Gain  Gain=miu1/m1
  Gain17 : Gain  Gain=-1
  Gain18 : Gain  Gain=-k2/m1
  Gain19 : Gain  Gain=miu2/m1
  Gain2 : Gain  Gain=miu2/m2
  Gain20 : Gain  Gain=C  Multiplication=Matrix(K*u)
  Gain21 : Gain  Gain=C  Multiplication=Matrix(K*u)
  Gain22 : Gain  Gain=L  Multiplication=Matrix(K*u)
  Gain3 : Gain  Gain=1/m2
  Gain4 : Gain  Gain=-delta1/m1
  Gain5 : Gain  Gain=-k1/m1
  Gain6 : Gain  Gain=miu1/m1
  Gain7 : Gain  Gain=-1
  Gain8 : Gain  Gain=-k2/m1
  Gain9 : Gain  Gain=miu2/m1
  Integrator : Integrator  InitialCondition=0.2
  Integrator1 : Integrator  InitialCondition=-0.1
  Integrator2 : Integrator  InitialCondition=0.2
  Integrator3 : Integrator  InitialCondition=0.3
  Integrator{4..7} (4 alike) : Integrator
  Math Function{,1..5} (6 alike) : Math  Operator=pow
  Mux : Mux
  Mux1 : Mux
  Scope : Scope  NumInputPorts=2
  Sum : Sum  Inputs=++++
  Sum1 : Sum  Inputs=++++
  Sum10 : Sum  Inputs=++|
  Sum2 : Sum  Inputs=++++++
  Sum3 : Sum  Inputs=++++++
  Sum4 : Sum  Inputs=|+-
  Sum5 : Sum  Inputs=|+-
  Sum6 : Sum  Inputs=+-
  Sum7 : Sum  Inputs=|++
  Sum8 : Sum  Inputs=|++
  Sum9 : Sum  Inputs=++|
  xhat : Outport
  wires:
  u1/1 -> Gain11/1
  Gain3/1 -> Sum7/1, Sum/1
  Mux/1 -> Scope/1, Gain21/1  "x"
  Gain4/1 -> Sum2/6
  Integrator/1 -> Gain/1, Integrator1/1, Mux/4  "x4"
  Sum4/1 -> Gain7/1, Math Function/1, Gain1/1  "x2-x1"
  Integrator3/1 -> Sum4/2, Math Function1/1, Gain5/1, Mux/1  "x1"
  Gain8/1 -> Sum2/3
  Gain7/1 -> Math Function2/1, Gain8/1  "x1-x2"
  Math Function2/1 -> Gain9/1
  Gain5/1 -> Sum2/5
  Gain1/1 -> Sum/3
  Constant2/1 -> Math Function2/2
  Gain9/1 -> Sum2/2
  Sum/1 -> Integrator/1  "x4dot"
  Math Function1/1 -> Gain6/1
  Gain/1 -> Sum/4
  Gain2/1 -> Sum/2
  Integrator1/1 -> Mux/2, Sum4/1  "x2"
  Constant/1 -> Math Function/2
  Math Function/1 -> Gain2/1
  Integrator2/1 -> Gain4/1, Integrator3/1, Mux/3  "x3"
  Gain6/1 -> Sum2/4
  u2/1 -> Gain3/1
  Sum2/1 -> Integrator2/1  "x3dot"
  Constant1/1 -> Math Function1/2
  Gain11/1 -> Sum8/1, Sum2/1
  Constant4/1 -> Math Function4/2
  Sum3/1 -> Integrator6/1  "x3dot"
  Gain16/1 -> Sum3/4
  Math Function3/1 -> Gain13/1
  Constant3/1 -> Math Function3/2
  Integrator5/1 -> Sum5/1, Mux1/2  "x2hat"
  Gain13/1 -> Sum1/2
  Gain10/1 -> Sum1/4
  Math Function4/1 -> Gain16/1
  Sum1/1 -> Integrator4/1  "x4dot"
  Gain19/1 -> Sum3/2
  Constant5/1 -> Math Function5/2
  Gain12/1 -> Sum1/3
  Gain15/1 -> Sum3/5
  Math Function5/1 -> Gain19/1
  Gain17/1 -> Gain18/1, Math Function5/1  "x1-x2"
  Gain18/1 -> Sum3/3
  Integrator7/1 -> Mux1/1, Gain15/1, Math Function4/1, Sum5/2  "x1hat"
  Sum5/1 -> Gain12/1, Math Function3/1, Gain17/1  "x2-x1"
  Gain14/1 -> Sum3/6
  Mux1/1 -> xhat/1, Scope/2, Gain20/1  "xhat"
  Gain20/1 -> Sum6/2
  Gain21/1 -> Sum6/1
  Sum6/1 -> Gain22/1
  Gain22/1 -> Demux/1
  Sum7/1 -> Sum1/1
  Sum8/1 -> Sum3/1
  Demux/4 -> Sum7/2
  Demux/3 -> Sum8/2
  Integrator4/1 -> Sum9/2
  Sum9/1 -> Mux1/4, Gain10/1, Integrator5/1  "x4hat"
  Demux/2 -> Sum9/1
  Integrator6/1 -> Sum10/2
  Sum10/1 -> Mux1/3, Gain14/1, Integrator7/1  "x3hat"
  Demux/1 -> Sum10/1

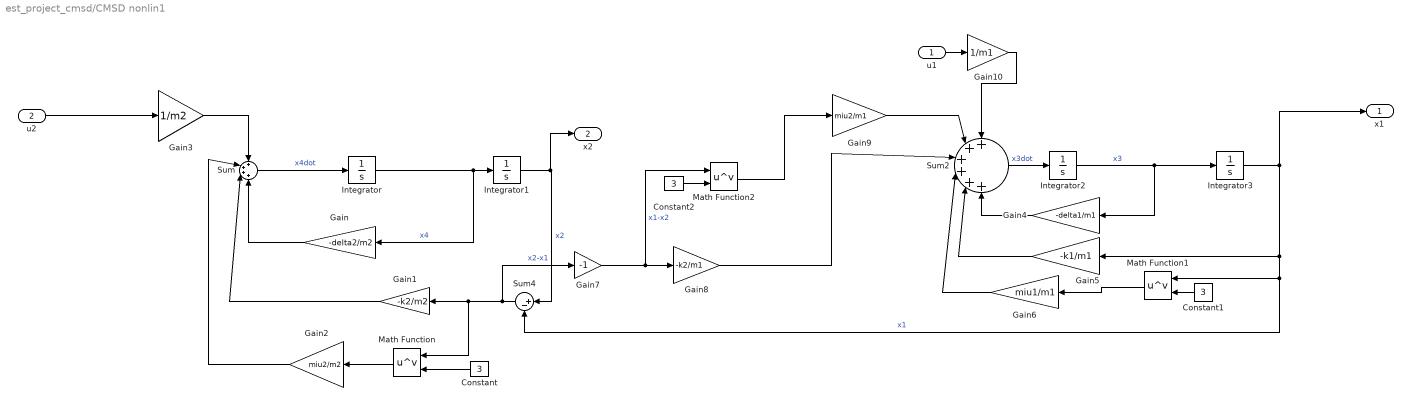
== system est_project_cmsd/CMSD nonlin1 ==
  u1 : Inport
  u2 : Inport  Port=2
  Constant : Constant  Value=3
  Constant1 : Constant  Value=3
  Constant2 : Constant  Value=3
  Gain : Gain  Gain=-delta2/m2
  Gain1 : Gain  Gain=-k2/m2
  Gain10 : Gain  Gain=1/m1
  Gain2 : Gain  Gain=miu2/m2
  Gain3 : Gain  Gain=1/m2
  Gain4 : Gain  Gain=-delta1/m1
  Gain5 : Gain  Gain=-k1/m1
  Gain6 : Gain  Gain=miu1/m1
  Gain7 : Gain  Gain=-1
  Gain8 : Gain  Gain=-k2/m1
  Gain9 : Gain  Gain=miu2/m1
  Integrator : Integrator  InitialCondition=0.2
  Integrator1 : Integrator  InitialCondition=0.3
  Integrator2 : Integrator  InitialCondition=0.4
  Integrator3 : Integrator  InitialCondition=0.1
  Math Function : Math  Operator=pow
  Math Function1 : Math  Operator=pow
  Math Function2 : Math  Operator=pow
  Sum : Sum  Inputs=++++
  Sum2 : Sum  Inputs=++++++
  Sum4 : Sum  Inputs=|+-
  x1 : Outport
  x2 : Outport  Port=2
  wires:
  Constant1/1 -> Math Function1/2
  Sum2/1 -> Integrator2/1  "x3dot"
  u2/1 -> Gain3/1
  Gain6/1 -> Sum2/4
  Integrator2/1 -> Integrator3/1, Gain4/1  "x3"
  Math Function/1 -> Gain2/1
  Constant/1 -> Math Function/2
  Integrator1/1 -> Sum4/1, x2/1  "x2"
  Gain2/1 -> Sum/2
  Gain/1 -> Sum/4
  Math Function1/1 -> Gain6/1
  Sum/1 -> Integrator/1  "x4dot"
  Gain9/1 -> Sum2/2
  Constant2/1 -> Math Function2/2
  Gain1/1 -> Sum/3
  Gain5/1 -> Sum2/5
  Gain3/1 -> Sum/1
  Math Function2/1 -> Gain9/1
  Gain7/1 -> Gain8/1, Math Function2/1  "x1-x2"
  Gain8/1 -> Sum2/3
  Integrator3/1 -> x1/1, Gain5/1, Math Function1/1, Sum4/2  "x1"
  Sum4/1 -> Gain1/1, Math Function/1, Gain7/1  "x2-x1"
  Integrator/1 -> Integrator1/1, Gain/1  "x4"
  Gain4/1 -> Sum2/6
  u1/1 -> Gain10/1
  Gain10/1 -> Sum2/1
